simulink model "RB_simblk"  (R2019b)
settings: Solver=VariableStepAuto  StartTime=0.0  StopTime=10.0  RelTol=1e-3
libraries: simulink x5
settings Model: Creator=Paresh  LastModifiedBy=Paresh

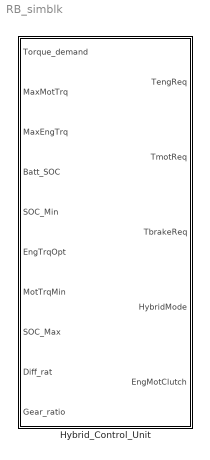
== system RB_simblk ==
  Hybrid_Control_Unit : Subsystem

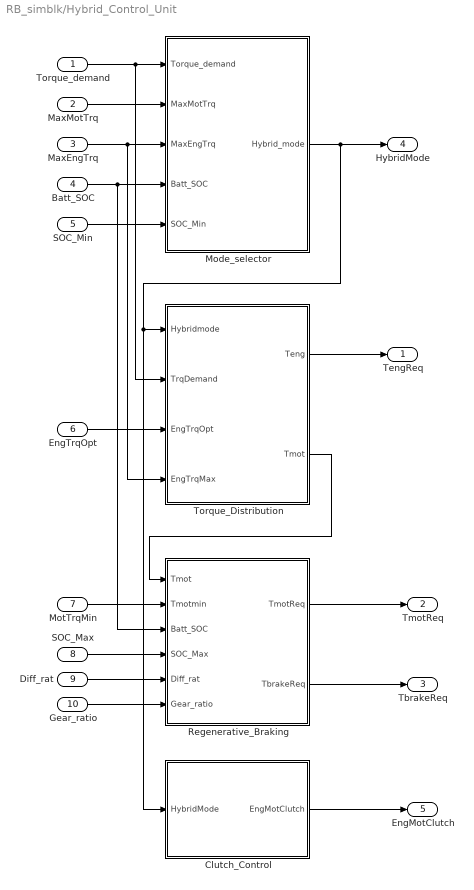
== system RB_simblk/Hybrid_Control_Unit ==
  Torque_demand : Inport
  MaxMotTrq : Inport  Port=2
  MaxEngTrq : Inport  Port=3
  Batt_SOC : Inport  Port=4
  SOC_Min : Inport  Port=5
  EngTrqOpt : Inport  Port=6
  MotTrqMin : Inport  Port=7
  SOC_Max : Inport  Port=8
  Diff_rat : Inport  Port=9
  Gear_ratio : Inport  Port=10
  Clutch_Control : Subsystem
  Mode_selector : Subsystem
  Regenerative_Braking : Subsystem
  Torque_Distribution : Subsystem
  TengReq : Outport
  TmotReq : Outport  Port=2
  TbrakeReq : Outport  Port=3
  HybridMode : Outport  Port=4
  EngMotClutch : Outport  Port=5
  wires:
  Torque_demand/1 -> Torque_Distribution/2(TrqDemand), Mode_selector/1(Torque_demand)
  MaxMotTrq/1 -> Mode_selector/2(MaxMotTrq)
  MaxEngTrq/1 -> Torque_Distribution/4(EngTrqMax), Mode_selector/3(MaxEngTrq)
  Batt_SOC/1 -> Regenerative_Braking/3(Batt_SOC), Mode_selector/4(Batt_SOC)
  SOC_Min/1 -> Mode_selector/5(SOC_Min)
  Mode_selector/1(Hybrid_mode) -> Clutch_Control/1(HybridMode), Torque_Distribution/1(Hybridmode), HybridMode/1
  Torque_Distribution/1(Teng) -> TengReq/1
  EngTrqOpt/1 -> Torque_Distribution/3(EngTrqOpt)
  Torque_Distribution/2(Tmot) -> Regenerative_Braking/1(Tmot)
  Regenerative_Braking/2(TbrakeReq) -> TbrakeReq/1
  Regenerative_Braking/1(TmotReq) -> TmotReq/1
  MotTrqMin/1 -> Regenerative_Braking/2(Tmotmin)
  SOC_Max/1 -> Regenerative_Braking/4(SOC_Max)
  Diff_rat/1 -> Regenerative_Braking/5(Diff_rat)
  Gear_ratio/1 -> Regenerative_Braking/6(Gear_ratio)
  Clutch_Control/1(EngMotClutch) -> EngMotClutch/1

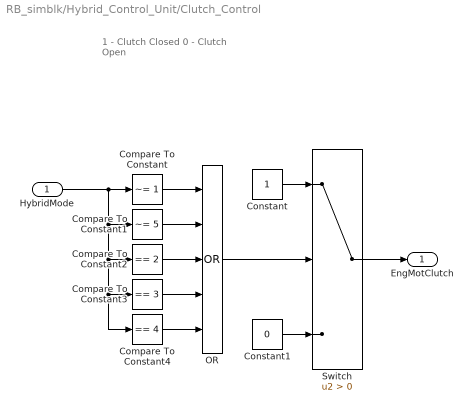
== system RB_simblk/Hybrid_Control_Unit/Clutch_Control ==
  note: 1 - Clutch Closed
      | 0 - Clutch Open
  HybridMode : Inport
  Compare To Constant : simulink/Logic and Bit Operations/Compare To Constant  relop=~=  const=1  OutDataTypeStr=boolean
  Compare To Constant1 : simulink/Logic and Bit Operations/Compare To Constant  relop=~=  const=5  OutDataTypeStr=boolean
  Compare To Constant2 : simulink/Logic and Bit Operations/Compare To Constant  relop===  const=2  OutDataTypeStr=boolean
  Compare To Constant3 : simulink/Logic and Bit Operations/Compare To Constant  relop===  const=3  OutDataTypeStr=boolean
  Compare To Constant4 : simulink/Logic and Bit Operations/Compare To Constant  relop===  const=4  OutDataTypeStr=boolean
  Constant : Constant
  Constant1 : Constant  Value=0
  OR : Logic  Operator=OR  Inputs=5  AllPortsSameDT=off  OutDataTypeStr=boolean
  Switch : Switch  Criteria=u2 > Threshold
  EngMotClutch : Outport
  wires:
  Switch/1 -> EngMotClutch/1
  Constant/1 -> Switch/1
  Constant1/1 -> Switch/3
  Compare To Constant/1 -> OR/1
  OR/1 -> Switch/2
  Compare To Constant1/1 -> OR/2
  Compare To Constant4/1 -> OR/5
  Compare To Constant3/1 -> OR/4
  Compare To Constant2/1 -> OR/3
  HybridMode/1 -> Compare To Constant4/1, Compare To Constant3/1, Compare To Constant2/1, Compare To Constant1/1, Compare To Constant/1

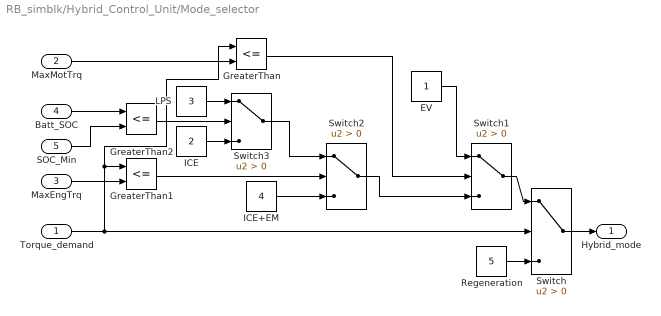
== system RB_simblk/Hybrid_Control_Unit/Mode_selector ==
  Torque_demand : Inport
  MaxMotTrq : Inport  Port=2
  MaxEngTrq : Inport  Port=3
  Batt_SOC : Inport  Port=4
  SOC_Min : Inport  Port=5
  EV : Constant
  GreaterThan : RelationalOperator  Operator=<=  OutDataTypeStr=boolean  RndMeth=Simplest
  GreaterThan1 : RelationalOperator  Operator=<=  OutDataTypeStr=boolean  RndMeth=Simplest
  GreaterThan2 : RelationalOperator  Operator=<=  OutDataTypeStr=boolean  RndMeth=Simplest
  ICE : Constant  Value=2
  ICE+EM : Constant  Value=4
  LPS : Constant  Value=3
  Regeneration : Constant  Value=5
  Switch{,1..3} (4 alike) : Switch  Criteria=u2 > Threshold
  Hybrid_mode : Outport
  wires:
  Torque_demand/1 -> GreaterThan/1, GreaterThan1/1, Switch/2
  Regeneration/1 -> Switch/3
  MaxMotTrq/1 -> GreaterThan/2
  GreaterThan/1 -> Switch1/2
  EV/1 -> Switch1/1
  Switch/1 -> Hybrid_mode/1
  MaxEngTrq/1 -> GreaterThan1/2
  GreaterThan1/1 -> Switch2/2
  Switch2/1 -> Switch1/3
  ICE+EM/1 -> Switch2/3
  Switch1/1 -> Switch/1
  Batt_SOC/1 -> GreaterThan2/1
  SOC_Min/1 -> GreaterThan2/2
  GreaterThan2/1 -> Switch3/2
  Switch3/1 -> Switch2/1
  ICE/1 -> Switch3/3
  LPS/1 -> Switch3/1

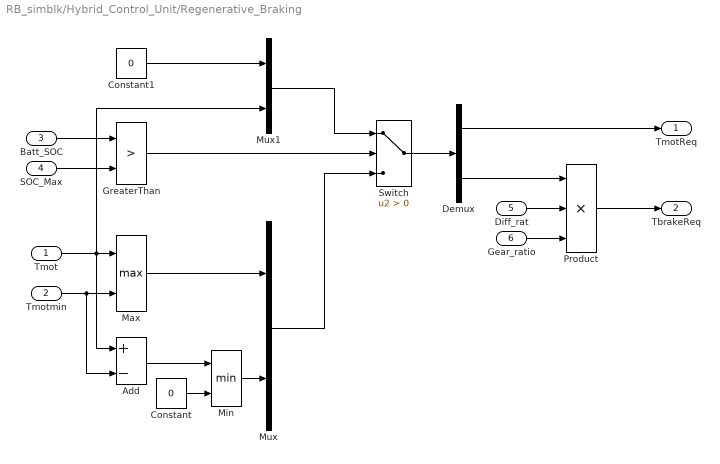
== system RB_simblk/Hybrid_Control_Unit/Regenerative_Braking ==
  Tmot : Inport
  Tmotmin : Inport  Port=2
  Batt_SOC : Inport  Port=3
  SOC_Max : Inport  Port=4
  Diff_rat : Inport  Port=5
  Gear_ratio : Inport  Port=6
  Add : Sum  Inputs=+-
  Constant : Constant  Value=0
  Constant1 : Constant  Value=0
  Demux : Demux  Outputs=2
  GreaterThan : RelationalOperator  Operator=>  OutDataTypeStr=boolean  RndMeth=Simplest
  Max : MinMax  Function=max  Inputs=2
  Min : MinMax  Inputs=2
  Mux : Mux  Inputs=2
  Mux1 : Mux  Inputs=2
  Product : Product  Inputs=3
  Switch : Switch  Criteria=u2 > Threshold
  TmotReq : Outport
  TbrakeReq : Outport  Port=2
  wires:
  Tmotmin/1 -> Add/2, Max/2
  Tmot/1 -> Mux1/2, Add/1, Max/1
  Constant/1 -> Min/2
  Add/1 -> Min/1
  Batt_SOC/1 -> GreaterThan/1
  SOC_Max/1 -> GreaterThan/2
  GreaterThan/1 -> Switch/2
  Min/1 -> Mux/2
  Max/1 -> Mux/1
  Mux/1 -> Switch/3
  Switch/1 -> Demux/1
  Demux/1 -> TmotReq/1
  Mux1/1 -> Switch/1
  Constant1/1 -> Mux1/1
  Gear_ratio/1 -> Product/3
  Diff_rat/1 -> Product/2
  Demux/2 -> Product/1
  Product/1 -> TbrakeReq/1

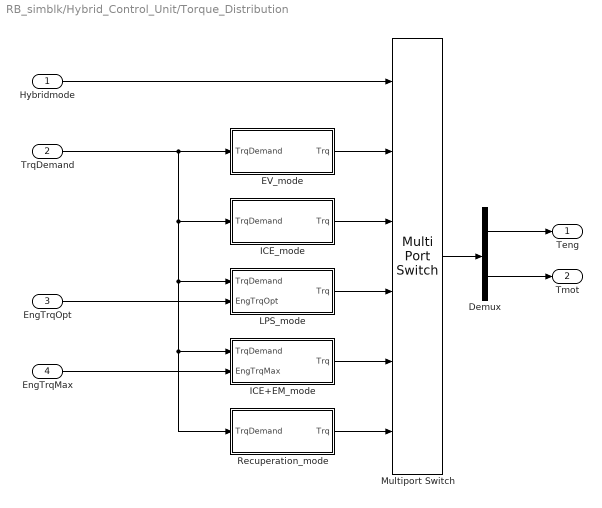
== system RB_simblk/Hybrid_Control_Unit/Torque_Distribution ==
  Hybridmode : Inport
  TrqDemand : Inport  Port=2
  EngTrqOpt : Inport  Port=3
  EngTrqMax : Inport  Port=4
  Demux : Demux  Outputs=2
  EV_mode : Subsystem
  ICE+EM_mode : Subsystem
  ICE_mode : Subsystem
  LPS_mode : Subsystem
  Multiport Switch : MultiPortSwitch  Inputs=5
  Recuperation_mode : Subsystem
  Teng : Outport
  Tmot : Outport  Port=2
  wires:
  Hybridmode/1 -> Multiport Switch/1
  Multiport Switch/1 -> Demux/1
  Demux/2 -> Tmot/1
  Demux/1 -> Teng/1
  EV_mode/1(Trq) -> Multiport Switch/2
  TrqDemand/1 -> Recuperation_mode/1(TrqDemand), ICE+EM_mode/1(TrqDemand), LPS_mode/1(TrqDemand), ICE_mode/1(TrqDemand), EV_mode/1(TrqDemand)
  EngTrqOpt/1 -> LPS_mode/2(EngTrqOpt)
  LPS_mode/1(Trq) -> Multiport Switch/4
  ICE_mode/1(Trq) -> Multiport Switch/3
  ICE+EM_mode/1(Trq) -> Multiport Switch/5
  Recuperation_mode/1(Trq) -> Multiport Switch/6
  EngTrqMax/1 -> ICE+EM_mode/2(EngTrqMax)

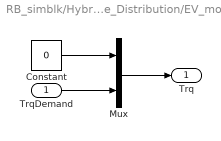
== system RB_simblk/Hybrid_Control_Unit/Torque_Distribution/EV_mode ==
  TrqDemand : Inport
  Constant : Constant  Value=0
  Mux : Mux  Inputs=2
  Trq : Outport
  wires:
  Mux/1 -> Trq/1
  Constant/1 -> Mux/1
  TrqDemand/1 -> Mux/2

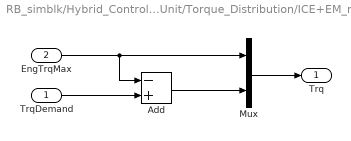
== system RB_simblk/Hybrid_Control_Unit/Torque_Distribution/ICE+EM_mode ==
  TrqDemand : Inport
  EngTrqMax : Inport  Port=2
  Add : Sum  Inputs=-+
  Mux : Mux  Inputs=2
  Trq : Outport
  wires:
  Add/1 -> Mux/2
  Mux/1 -> Trq/1
  EngTrqMax/1 -> Add/1, Mux/1
  TrqDemand/1 -> Add/2

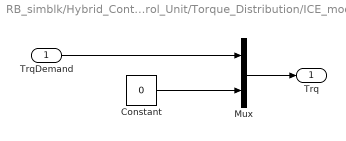
== system RB_simblk/Hybrid_Control_Unit/Torque_Distribution/ICE_mode ==
  TrqDemand : Inport
  Constant : Constant  Value=0
  Mux : Mux  Inputs=2
  Trq : Outport
  wires:
  Mux/1 -> Trq/1
  TrqDemand/1 -> Mux/1
  Constant/1 -> Mux/2

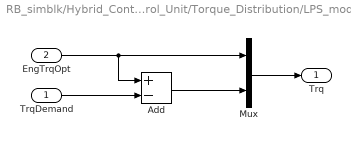
== system RB_simblk/Hybrid_Control_Unit/Torque_Distribution/LPS_mode ==
  TrqDemand : Inport
  EngTrqOpt : Inport  Port=2
  Add : Sum  Inputs=+-
  Mux : Mux  Inputs=2
  Trq : Outport
  wires:
  EngTrqOpt/1 -> Add/1, Mux/1
  Mux/1 -> Trq/1
  TrqDemand/1 -> Add/2
  Add/1 -> Mux/2

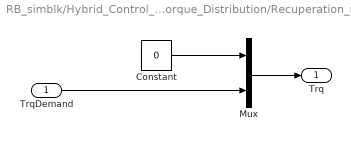
== system RB_simblk/Hybrid_Control_Unit/Torque_Distribution/Recuperation_mode ==
  TrqDemand : Inport
  Constant : Constant  Value=0
  Mux : Mux  Inputs=2
  Trq : Outport
  wires:
  Mux/1 -> Trq/1
  TrqDemand/1 -> Mux/2
  Constant/1 -> Mux/1
